simulink model "EKF_AnchorEstimate"  (R2015b)
settings: Solver=VariableStepAuto  SolverMode=SingleTasking  StartTime=0.0  StopTime=5000  FixedStep=0.01  MaxStep=0.01  RelTol=1e-3
values from neighbouring files (symbols this model uses):
  anchor_pos = [0 0 0 ... (first row only)    [script.m]
  dt = 0.1    [script.m]
  dtDeca = 0.3    [script.m]
  Q = zeros(length(xhat),length(xhat))    [script.m]
  RDeca = 0.0025    [script.m]
libraries: simulink x1
settings Model: Creator=Phil Goddard  LastModifiedBy=mathias
settings DataIOCC: SaveFormat=Array  SignalLoggingSaveFormat=ModelDataLogs
settings OptimizationCC: ExpressionDepthLimit=2147483647
settings DebuggingCC: UnderspecifiedInitializationDetection=Classic  MergeDetectMultiDrivingBlocksExec=none  SolverPrmCheckMsg=warning  FcnCallInpInsideContextMsg=UseLocalSettings  StateNameClashWarn=warning
settings HardwareCC: ProdBitPerPointer=32  ProdLargestAtomicFloat=None  ProdIntDivRoundTo=Undefined  ProdEndianess=Unspecified  ProdWordSize=32  ProdHWDeviceType=32-bit Generic
settings SFSimCC: SimParseCustomCode=off
settings GRTTargetCC: GeneratePreprocessorConditionals=Disable all  CombineOutputUpdateFcns=off  GRTInterface=on
settings ConfigComp: CovModelRefEnable=Off

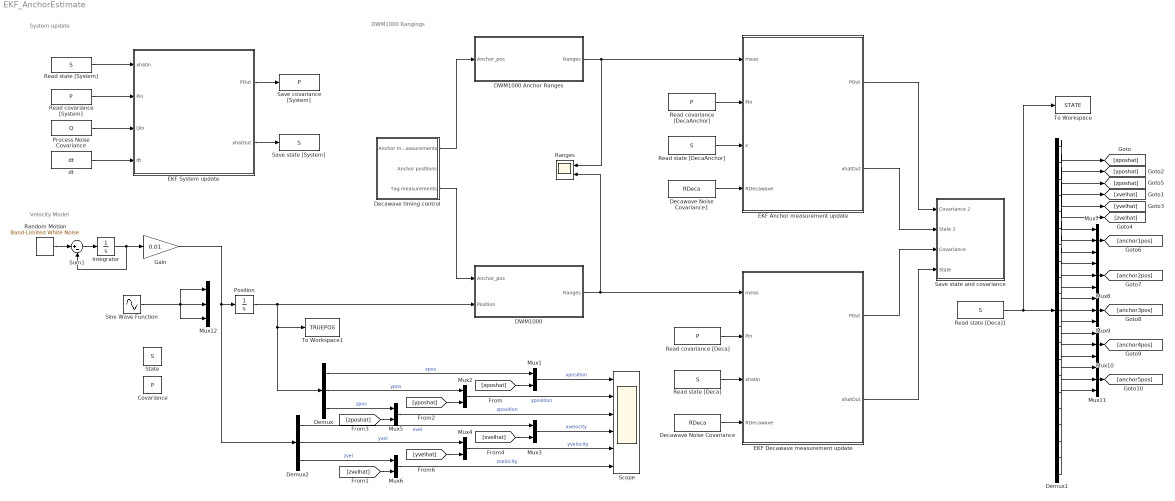
== system EKF_AnchorEstimate ==
  note: System update
  note: DWM1000 Rangings
  note: Velocity Model
  Covariance : DataStoreMemory  DataStoreName=P  ReadBeforeWriteMsg=warning  WriteAfterWriteMsg=warning  WriteAfterReadMsg=warning  InitialValue=P
  "DWM1000 " : MATLAB Function  TreatAsAtomicUnit=on  SystemSampleTime=dtDeca
  DWM1000 Anchor Ranges : MATLAB Function  TreatAsAtomicUnit=on  SystemSampleTime=dtDeca
  Decawave Noise Covariance : Constant  Value=RDeca
  Decawave Noise Covariance1 : Constant  Value=RDeca
  Decawave timing control : Subsystem  mask{Ratio=20}
      mask DialogControl Control2 Prompt: Ratio between Tag and Achor measurements
  Demux : Demux  Outputs=3
  Demux1 : Demux  Outputs=21
  Demux2 : Demux  Outputs=3
  EKF Anchor measurement update : MATLAB Function  TreatAsAtomicUnit=on
  EKF Decawave measurement update : MATLAB Function  TreatAsAtomicUnit=on
  EKF System update : MATLAB Function  TreatAsAtomicUnit=on  SystemSampleTime=dt
  Gain : Gain  Gain=0.01
  Integrator : Integrator
  Mux{1..6} (6 alike) : Mux  Inputs=2
  Mux{7..12} (6 alike) : Mux  Inputs=3
  Position : Integrator  InitialCondition=[1; 1; 1]
  Process Noise Covariance : Constant  Value=Q
  Random Motion : simulink/Sources/Band-Limited White Noise  Cov=[1; 0.4; 0.01]  Ts=0.01  seed=[23341]
  Ranges : Scope  NumInputPorts=2
  Read covariance [DecaAnchor] : DataStoreRead  DataStoreName=P
  Read covariance [Deca] : DataStoreRead  DataStoreName=P
  Read covariance [System] : DataStoreRead  DataStoreName=P  SampleTime=dt
  Read state [DecaAnchor] : DataStoreRead  DataStoreName=S
  Read state [Deca] : DataStoreRead  DataStoreName=S
  Read state [Deca]1 : DataStoreRead  DataStoreName=S
  Read state [System] : DataStoreRead  DataStoreName=S  SampleTime=dt
  Save covariance [System] : DataStoreWrite  DataStoreName=P
  Save state [System] : DataStoreWrite  DataStoreName=S
  Save state and covariance : Subsystem
  Scope : Scope  NumInputPorts=6
  Sine Wave Function : Sin  Amplitude=0.001  Frequency=0.01  SampleTime=0
  State : DataStoreMemory  DataStoreName=S  ReadBeforeWriteMsg=warning  WriteAfterWriteMsg=warning  WriteAfterReadMsg=warning  InitialValue=xhat
  Sum1 : Sum  Inputs=|+-
  To Workspace : ToWorkspace  VariableName=STATE  SaveFormat=Timeseries  SampleTime=-1
  To Workspace1 : ToWorkspace  VariableName=TRUEPOS  SaveFormat=Timeseries  SampleTime=dt
  dt : Constant  Value=dt
  wires:
  Integrator/1 -> Gain/1, Sum1/2
  Demux/1 -> Mux1/1  "xpos"
  Demux/2 -> Mux2/1  "ypos"
  Mux1/1 -> Scope/1  "xposition"
  [xposhat] -> Mux1/2
  [yposhat] -> Mux2/2
  Mux2/1 -> Scope/2  "yposition"
  [xvelhat] -> Mux3/2
  Demux2/1 -> Mux3/1  "xvel"
  Mux3/1 -> Scope/4  "xvelocity"
  [yvelhat] -> Mux4/2
  Demux2/2 -> Mux4/1  "yvel"
  Mux4/1 -> Scope/5  "yvelocity"
  Mux5/1 -> Scope/3  "zposition"
  Demux/3 -> Mux5/1  "zpos"
  Mux6/1 -> Scope/6  "zvelocity"
  Demux2/3 -> Mux6/1  "zvel"
  [zvelhat] -> Mux6/2
  [zposhat] -> Mux5/2
  Random Motion/1 -> Sum1/1
  Sum1/1 -> Integrator/1
  Read covariance [Deca]/1 -> EKF Decawave measurement update/2(PIn)
  Decawave Noise Covariance/1 -> EKF Decawave measurement update/4(RDecawave)
  Read state [Deca]/1 -> EKF Decawave measurement update/3(xhatIn)
  Read covariance [DecaAnchor]/1 -> EKF Anchor measurement update/2(PIn)
  Decawave Noise Covariance1/1 -> EKF Anchor measurement update/4(RDecawave)
  Read state [DecaAnchor]/1 -> EKF Anchor measurement update/3(x)
  DWM1000 Anchor Ranges/1(Ranges) -> Ranges/1, EKF Anchor measurement update/1(meas)
  "DWM1000 "/1(Ranges) -> EKF Decawave measurement update/1(meas), Ranges/2
  Position/1 -> "DWM1000 "/2(Position), Demux/1, To Workspace1/1
  EKF System update/2(xhatOut) -> Save state [System]/1
  Read state [System]/1 -> EKF System update/1(xhatIn)
  dt/1 -> EKF System update/4(dt)
  EKF System update/1(POut) -> Save covariance [System]/1
  Process Noise Covariance/1 -> EKF System update/3(Qin)
  Read covariance [System]/1 -> EKF System update/2(Pin)
  Decawave timing control/3(Tag measurements) -> "DWM1000 "/1(Anchor_pos)
  Decawave timing control/1(Anchor measurements) -> DWM1000 Anchor Ranges/1(Anchor_pos)
  Demux1/1 -> [xposhat]
  Demux1/4 -> [xvelhat]
  Demux1/2 -> [yposhat]
  Demux1/5 -> [yvelhat]
  Demux1/6 -> [zvelhat]
  Demux1/3 -> [zposhat]
  Demux1/7 -> Mux7/1
  Demux1/8 -> Mux7/2
  Demux1/9 -> Mux7/3
  Mux7/1 -> [anchor1pos]
  Mux8/1 -> [anchor2pos]
  Mux9/1 -> [anchor3pos]
  Demux1/11 -> Mux8/2
  Demux1/10 -> Mux8/1
  Demux1/13 -> Mux9/1
  Demux1/12 -> Mux8/3
  Demux1/14 -> Mux9/2
  Demux1/15 -> Mux9/3
  Mux10/1 -> [anchor4pos]
  Mux11/1 -> [anchor5pos]
  Demux1/16 -> Mux10/1
  Demux1/18 -> Mux10/3
  Demux1/17 -> Mux10/2
  Demux1/20 -> Mux11/2
  Demux1/21 -> Mux11/3
  Demux1/19 -> Mux11/1
  Read state [Deca]1/1 -> To Workspace/1, Demux1/1
  EKF Anchor measurement update/1(POut) -> Save state and covariance/1(Covariance 2)
  EKF Anchor measurement update/2(xhatOut) -> Save state and covariance/2(State 2)
  EKF Decawave measurement update/1(POut) -> Save state and covariance/3(Covariance)
  EKF Decawave measurement update/2(xhatOut) -> Save state and covariance/4(State)
  Sine Wave Function/1 -> Mux12/3, Mux12/1, Mux12/2
  Gain/1 -> Demux2/1, Position/1

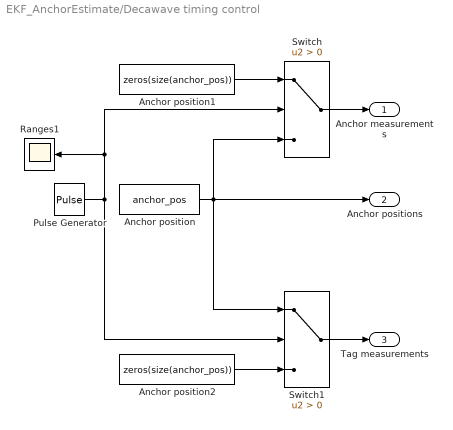
== system EKF_AnchorEstimate/Decawave timing control ==
  Anchor position : Constant  Value=anchor_pos
  Anchor position1 : Constant  Value=zeros(size(anchor_pos))
  Anchor position2 : Constant  Value=zeros(size(anchor_pos))
  Pulse Generator : DiscretePulseGenerator  Period=Ratio  PulseWidth=Ratio-1  PhaseDelay=1  SampleTime=dtDeca
  Ranges1 : Scope
  Switch : Switch  Criteria=u2 > Threshold
  Switch1 : Switch  Criteria=u2 > Threshold
  Anchor measurements : Outport
  Anchor positions : Outport  Port=2
  Tag measurements : Outport  Port=3
  wires:
  Anchor position1/1 -> Switch/1
  Switch1/1 -> Tag measurements/1
  Anchor position/1 -> Switch/3, Anchor positions/1, Switch1/1
  Switch/1 -> Anchor measurements/1
  Anchor position2/1 -> Switch1/3
  Pulse Generator/1 -> Ranges1/1, Switch/2, Switch1/2

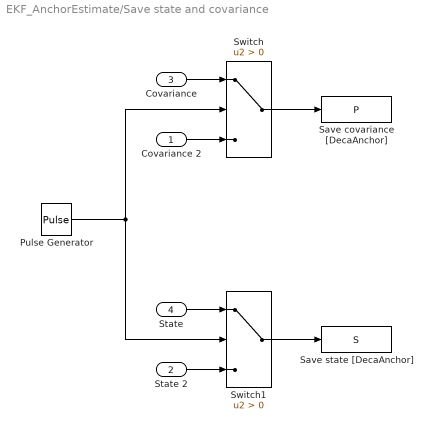
== system EKF_AnchorEstimate/Save state and covariance ==
  Covariance 2 : Inport
  State 2 : Inport  Port=2
  Covariance : Inport  Port=3
  State : Inport  Port=4
  Pulse Generator : DiscretePulseGenerator  Period=20  PulseWidth=19  PhaseDelay=1  SampleTime=dtDeca
  Save covariance [DecaAnchor] : DataStoreWrite  DataStoreName=P
  Save state [DecaAnchor] : DataStoreWrite  DataStoreName=S
  Switch : Switch  Criteria=u2 > Threshold
  Switch1 : Switch  Criteria=u2 > Threshold
  wires:
  State/1 -> Switch1/1
  Covariance 2/1 -> Switch/3
  Covariance/1 -> Switch/1
  Switch1/1 -> Save state [DecaAnchor]/1
  State 2/1 -> Switch1/3
  Pulse Generator/1 -> Switch1/2, Switch/2
  Switch/1 -> Save covariance [DecaAnchor]/1

== matlab function EKF_AnchorEstimate/DWM1000  ==
  data: Ranges output; Anchor_pos input; Position input double
function Ranges   = DWM1000(Anchor_pos, Position)


persistent noiseSeed R

if isempty(R)
    R = zeros(size(Anchor_pos,1), 1);
end

noiseVar = 0.0025;

if any(Anchor_pos(:))

    if isempty(noiseSeed)
        noiseSeed = 1;
    end

    rng(noiseSeed);

    devices = size(Anchor_pos,1);

    R = zeros(devices,1);

    for n=1:devices
        R(n) = sqrt( (Anchor_pos(n,1)-Position(1))^2 + (Anchor_pos(n,2)-Position(2))^2 + (Anchor_pos(n,3)-Position(3))^2 ) + sqrt(noiseVar).*randn();
    end

    noiseSeed = noiseSeed + 13;

end

Ranges = R;

== matlab function EKF_AnchorEstimate/EKF Decawave measurement update ==
  data: POut output; xhatOut output double; meas input double; PIn input; xhatIn input; RDecawave input
function [POut, xhatOut] = DecaMeasurementUpdate(meas, PIn, xhatIn, RDecawave)

devices = size(meas,1);

yhat = zeros(devices,1); 
H = zeros(devices,size(xhatIn,1)); 
for n=1:devices
    ind = 6 + (n-1)*3;
    yhat(n) = sqrt( (xhatIn(ind+1)-xhatIn(1))^2 + (xhatIn(ind+2)-xhatIn(2))^2 + (xhatIn(ind+3)-xhatIn(3))^2 );
    H(n,1) = -(xhatIn(ind+1) - xhatIn(1))/yhat(n); 
    H(n,2) = -(xhatIn(ind+2) - xhatIn(2))/yhat(n);
    H(n,3) = -(xhatIn(ind+3) - xhatIn(3))/yhat(n);
    
    H(n,ind+1) = (xhatIn(ind+1) - xhatIn(1))/yhat(n); 
    H(n,ind+2) = (xhatIn(ind+2) - xhatIn(2))/yhat(n);
    H(n,ind+3) = (xhatIn(ind+3) - xhatIn(3))/yhat(n);
end


% Calculate the Kalman gain
K = PIn*H'/(H*PIn*H' + eye(devices).*RDecawave);

% Update the state and covariance estimates
xhatOut = xhatIn + K*(meas - yhat);
POut = (eye(size(K,1))-K*H)*PIn;

== matlab function EKF_AnchorEstimate/EKF System update ==
  data: xhatIn input; Pin input; POut output; Qin input; xhatOut output double; dt input double
function [POut, xhatOut] = SystemUpdate(xhatIn, Pin, Qin, dt)


F = eye(length(xhatIn));
 
F(1,4) = dt;
F(2,5) = dt;
F(3,6) = dt;

% Propogate the state and covariance matrices
xhatOut = F*xhatIn;
POut = F*Pin*F' + Qin;

== matlab function EKF_AnchorEstimate/DWM1000 Anchor Ranges ==
  data: Ranges output; Anchor_pos input
function Ranges = DWM1000_ANCHOR(Anchor_pos)

persistent noiseSeed R

if isempty(R)
    N = size(Anchor_pos,1);
    R = zeros((N-1)*N/2, 1);
end

noiseVar = 0.0025;

if any(Anchor_pos(:))

    if isempty(noiseSeed)
        noiseSeed = 1;
    end

    rng(noiseSeed);

    N = size(Anchor_pos,1);

    R = zeros((N-1)*N/2,1);

    Rcnt = 1;
    %h_anchor = zeros((N-1)*N/2, 1);
    cnt = N;
    for n = 1:N
        for j = 1:cnt-1
            ind2 = n + j;
            R(Rcnt) = sqrt( (Anchor_pos(n,1)-Anchor_pos(ind2,1))^2 + (Anchor_pos(n,2)-Anchor_pos(ind2,2))^2 + (Anchor_pos(n,3)-Anchor_pos(ind2,3))^2 )  + sqrt(noiseVar).*randn();
            Rcnt = Rcnt + 1;
        end
        cnt = cnt - 1;
    end

    noiseSeed = noiseSeed + 13;

end

Ranges = R;

== matlab function EKF_AnchorEstimate/EKF Anchor measurement update ==
  data: POut output; xhatOut output double; meas input double; PIn input; x input; RDecawave input
function [POut, xhatOut] = DecaAnchorUpdate(meas, PIn, x, RDecawave)

N = length(meas);

devices = sqrt(2*N+1/4)+0.5;

Rcnt =  1;
yhat = zeros(N, 1);

ymeas = meas;


% This needs to be made variable-sized!
H = zeros(N, length(x));
cnt = devices;
for n = 1:devices
    ind1 = length(x)-(devices*3) + (n-1)*3;
    for j = 1:cnt-1
        ind2 = ind1 + 3*j;
        
        yhat(Rcnt) = sqrt( (x(ind1+1) - x(ind2+1))^2 + (x(ind1+2) - x(ind2+2))^2 + (x(ind1+3) - x(ind2+3))^2);
        H(Rcnt,ind1+1) = (x(ind1+1) - x(ind2+1))/yhat(Rcnt);
        H(Rcnt,ind2+1) = -(x(ind1+1) - x(ind2+1))/yhat(Rcnt);
        H(Rcnt,ind1+2) = (x(ind1+2) - x(ind2+2))/yhat(Rcnt);
        H(Rcnt,ind2+2) = -(x(ind1+2) - x(ind2+2))/yhat(Rcnt);
        H(Rcnt,ind1+3) = (x(ind1+3) - x(ind2+3))/yhat(Rcnt);
        H(Rcnt,ind2+3) = -(x(ind1+3) - x(ind2+3))/yhat(Rcnt);
        
        Rcnt = Rcnt + 1;
    end
    
    cnt = cnt - 1;
end

% Pin first device to [0 0 0]
H = [H; zeros(3,6) eye(3), zeros(3, length(x)-9)];
ymeas = [ymeas; 0; 0; 0];
yhat = [yhat; x(7); x(8); x(9)];

% Pin second device to [d 0 0]
H = [H; zeros(2,10) eye(2), zeros(2, length(x)-12)];
ymeas = [ymeas; 0; 0];
yhat = [yhat; x(11); x(12)];

% Pin third device to [d d 0]
H = [H; zeros(1,14) eye(1), zeros(1, length(x)-15)];
ymeas = [ymeas; 0];
yhat = [yhat; x(15)];

R = diag([diag(eye(N).*RDecawave)' 0 0 0 0 0 0]);

res = ymeas - yhat;

% Calculate the Kalman gain
K = PIn*H'/(H*PIn*H' + R);

% Update the state and covariance estimates
xhatOut = x + K*res;
POut = (eye(size(K,1))-K*H)*PIn;
